simulink model "Boost_Converter_Model"  (R2020a)
settings: Solver=VariableStepAuto  StartTime=0.0  StopTime=1  RelTol=1e-3
libraries: powerlib x13, powerlib_meascontrol x1
settings Model: Creator=Ricardo Romero  LastModifiedBy=Ricardo Romero

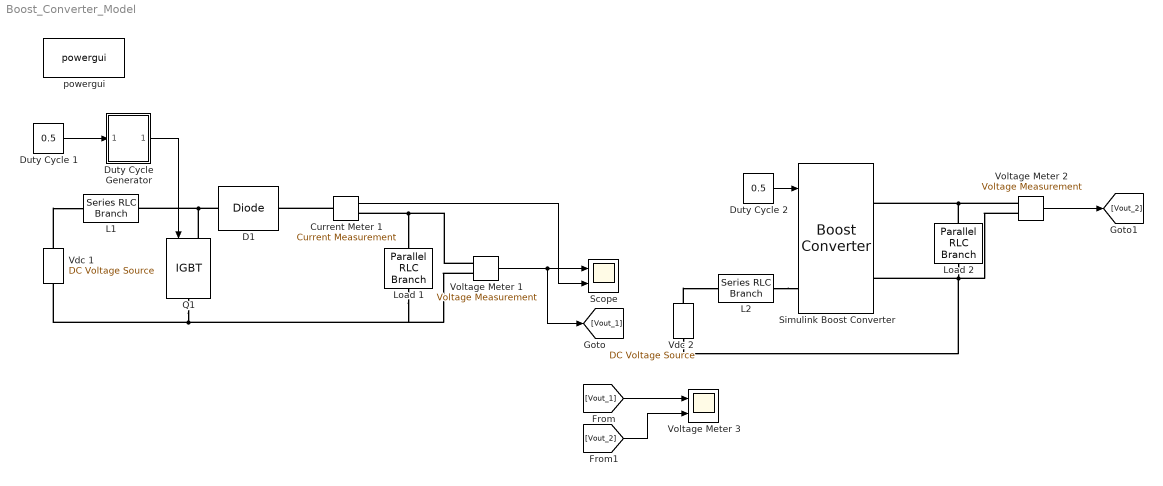
== system Boost_Converter_Model ==
  Current Meter 1 : powerlib/Measurements/Current Measurement  PhasorSimulation=off  OutputType=Complex  PSBequivalent=0
  D1 : powerlib/Power Electronics/Diode  Ron=0.001  Lon=0  Vf=0.8  IC=0  UseSnubber=0  Rs=500  Cs=250e-9  Measurements=off
  Duty Cycle Generator : Subsystem
  Duty Cycle 1 : Constant  Value=0.5
  Duty Cycle 2 : Constant  Value=0.5
  L1 : powerlib/Elements/Series RLC Branch  LConnTagsString=__new0  RConnTagsString=__new0  BranchType=L  Resistance=1  Inductance=1e-3  SetiL0=off  InitialCurrent=0  Capacitance=1e-6  Setx0=off  InitialVoltage=0  Measurements=None
  L2 : powerlib/Elements/Series RLC Branch  LConnTagsString=__new0  RConnTagsString=__new0  BranchType=L  Resistance=1  Inductance=1e-3  SetiL0=off  InitialCurrent=0  Capacitance=1e-6  Setx0=off  InitialVoltage=0  Measurements=None
  Load 1 : powerlib/Elements/Parallel RLC Branch  LConnTagsString=a  RConnTagsString=__new0  BranchType=RC  Resistance=10  Inductance=1e-3  SetiL0=off  InitialCurrent=0  Capacitance=20e-3  Setx0=off  InitialVoltage=0  Measurements=None
  Load 2 : powerlib/Elements/Parallel RLC Branch  LConnTagsString=a  RConnTagsString=__new0  BranchType=RC  Resistance=10  Inductance=1e-3  SetiL0=off  InitialCurrent=0  Capacitance=20e-3  Setx0=off  InitialVoltage=0  Measurements=None
  Q1 : powerlib/Power Electronics/IGBT  Ron=0.001  Lon=0  Vf=1  Tf=1e-6  Tt=2e-6  IC=0  Rs=1e5  Cs=inf  Measurements=off
  Scope : Scope  NumInputPorts=2
  Simulink Boost Converter : powerlib/Power Electronics/Boost Converter  ModelType=Average model (D-controlled)  Ron=1e-3  Rs=1e6  Cs=inf  Vforward=[0,0]  Ron_Diode=1e-3  Rs_Diode=1e6  Cs_Diode=inf  Vf_Diode=1e-3  Rs_CurrentSource=inf
      settings: SourceProductBaseCode=PS
  "Vdc 1 " : powerlib/Electrical Sources/DC Voltage Source  Amplitude=10  Measurements=None
  Vdc 2 : powerlib/Electrical Sources/DC Voltage Source  Amplitude=10  Measurements=None
  Voltage Meter 1 : powerlib/Measurements/Voltage Measurement  PhasorSimulation=off  OutputType=Complex  PSBequivalent=0
  Voltage Meter 2 : powerlib/Measurements/Voltage Measurement  PhasorSimulation=off  OutputType=Complex  PSBequivalent=0
  Voltage Meter 3 : Scope  NumInputPorts=2
  powergui : powerlib/powergui  Priority=1  SimulationMode=Discrete  SampleTime=5e-6  frequency=60  Iterations=50  frequencyindice=0  Pbase=100e6  ErrMax=1e-4  UnitsV=kV  UnitsW=MW  buscounter=0  FunctionMessages=off  echomessages=off  EnableUseOfTLC=off  CurrentSourceSwitches=off  DisableSnubberDevices=off  DisableRonSwitches=off  DisableVfSwitches=off  DisplayEquations=off  AutomaticDiscreteSolvers=off  SolverType=Tustin/Backward Euler (TBE)  Interpol=off  ExternalGateDelay=off  methode=off  Ts=100  x0status=blocks  SPID=on  SwTol=0  HookPort=off  NonlinearTolerance=1e-4  nMaxIteration=100  ContinueOnMaxIteration=off  RestoreLinks=warning  ResistiveCurrentMeasurement=off  Frange=[0:2:500]  Ylog=off  Xlog=on  ShowGrid=off  save=off  variable=ZData  structure=0  ZoomFFT=off  StartTime=0.0  cycles=1  DisplayStyle=1  fundamental=60  FreqAxis=off  MaxFrequency=1000  frequencyindicesteady=1  RmsSteady=1  display=off
  wires:
  Voltage Meter 1/1 -> [Vout_1], Scope/1
  Current Meter 1/1 -> Scope/2
  Duty Cycle 1/1 -> Duty Cycle Generator/1(In1)
  Duty Cycle Generator/1(Out1) -> Q1/1
  Duty Cycle 2/1 -> Simulink Boost Converter/1
  Voltage Meter 2/1 -> [Vout_2]
  [Vout_1] -> Voltage Meter 3/1
  [Vout_2] -> Voltage Meter 3/2
  connections:
  "Vdc 1 "/RConn1 -- L1/LConn1
  Q1/LConn1 -- L1/RConn1 -- D1/LConn1
  Q1/RConn1 -- Load 1/RConn1 -- Voltage Meter 1/LConn2 -- "Vdc 1 "/LConn1
  Current Meter 1/LConn1 -- D1/RConn1
  Voltage Meter 1/LConn1 -- Load 1/LConn1 -- Current Meter 1/RConn1
  L2/RConn1 -- Simulink Boost Converter/LConn1
  Vdc 2/RConn1 -- L2/LConn1
  Vdc 2/LConn1 -- Simulink Boost Converter/RConn2 -- Voltage Meter 2/LConn2 -- Load 2/RConn1
  Load 2/LConn1 -- Voltage Meter 2/LConn1 -- Simulink Boost Converter/RConn1

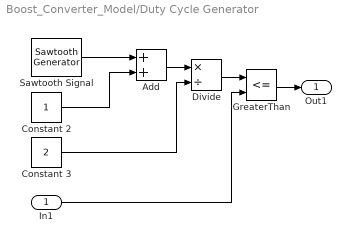
== system Boost_Converter_Model/Duty Cycle Generator ==
  In1 : Inport
  Add : Sum
  Constant 2 : Constant
  Constant 3 : Constant  Value=2
  Divide : Product  Inputs=*/
  GreaterThan : RelationalOperator  Operator=<=  OutDataTypeStr=boolean  RndMeth=Simplest
  Sawtooth Signal : powerlib_meascontrol/Pulse & Signal Generators/Sawtooth Generator  Freq=5e3  Phase=0  Ts=0
  Out1 : Outport
  wires:
  Divide/1 -> GreaterThan/1
  GreaterThan/1 -> Out1/1
  Constant 3/1 -> Divide/2
  Sawtooth Signal/1 -> Add/1
  Add/1 -> Divide/1
  Constant 2/1 -> Add/2
  In1/1 -> GreaterThan/2
